simulink model "blockModel"  (R2019b)
settings: Solver=VariableStepAuto  StartTime=0.0  StopTime=10.0  RelTol=1e-3
undefined symbols (not defined in the file or in its folder): gearbox, motor, tyre, veh
libraries: dspsigops x1
settings Model: Creator=picku  LastModifiedBy=picku

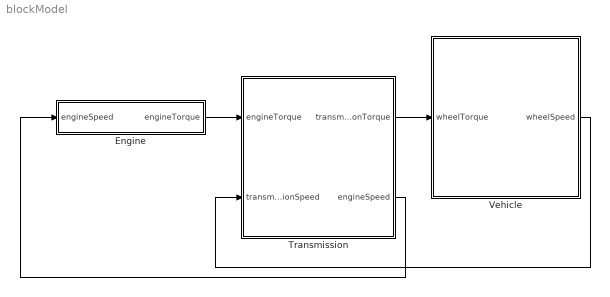
== system blockModel ==
  "Engine " : Subsystem
  Transmission : Subsystem
  Vehicle : Subsystem
  wires:
  Vehicle/1(wheelSpeed) -> Transmission/2(transmissionSpeed)
  Transmission/1(transmissionTorque) -> Vehicle/1(wheelTorque)
  "Engine "/1(engineTorque) -> Transmission/1("engineTorque ")
  Transmission/2(engineSpeed) -> "Engine "/1(engineSpeed)

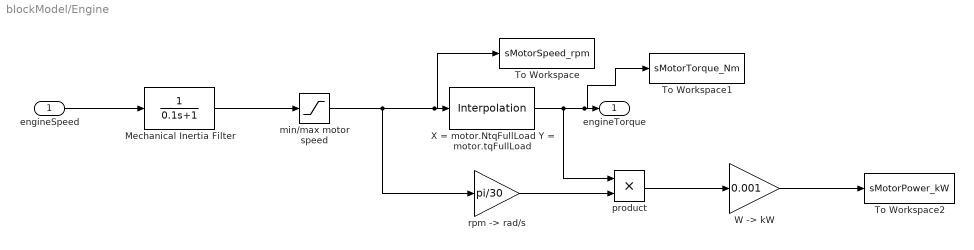
== system blockModel/Engine  ==
  engineSpeed : Inport
  Mechanical Inertia Filter : TransferFcn  Denominator=[0.1 1]
  To Workspace : ToWorkspace  VariableName=sMotorSpeed_rpm  SaveFormat=Timeseries  SampleTime=-1
  To Workspace1 : ToWorkspace  VariableName=sMotorTorque_Nm  SaveFormat=Timeseries  SampleTime=-1
  To Workspace2 : ToWorkspace  VariableName=sMotorPower_kW  SaveFormat=Timeseries  SampleTime=-1
  "W -> kW" : Gain  Gain=0.001
  X = motor.NtqFullLoad Y = motor.tqFullLoad : dspsigops/Interpolation  InterpSource=Specify via dialog  InterpPoints=[motor.NtqFullLoad' motor.tqFullLoad']  InterpMode=Linear  InterpL=3  InterpR=3  InterpAlpha=0.5  InvalidMode=Clip
      settings: SourceProductName=DSP System Toolbox  SourceProductBaseCode=DS
  min/max motor speed : Saturate  UpperLimit=motor.Nmax  LowerLimit=motor.Nmin
  product : Product
  "rpm -> rad/s" : Gain  Gain=pi/30
  engineTorque : Outport
  wires:
  min/max motor speed/1 -> X = motor.NtqFullLoad Y = motor.tqFullLoad/1, To Workspace/1, "rpm -> rad/s"/1
  X = motor.NtqFullLoad Y = motor.tqFullLoad/1 -> To Workspace1/1, engineTorque/1, product/1
  product/1 -> "W -> kW"/1
  "W -> kW"/1 -> To Workspace2/1
  Mechanical Inertia Filter/1 -> min/max motor speed/1
  "rpm -> rad/s"/1 -> product/2
  engineSpeed/1 -> Mechanical Inertia Filter/1

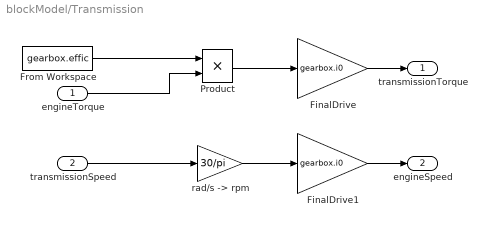
== system blockModel/Transmission ==
  "engineTorque " : Inport
  transmissionSpeed : Inport  Port=2
  FinalDrive : Gain  Gain=gearbox.i0
  FinalDrive1 : Gain  Gain=gearbox.i0
  From Workspace : FromWorkspace  VariableName=gearbox.effic  SampleTime=0
  "Product " : Product
  "rad/s -> rpm" : Gain  Gain=30/pi
  transmissionTorque : Outport
  engineSpeed : Outport  Port=2
  wires:
  "Product "/1 -> FinalDrive/1
  FinalDrive1/1 -> engineSpeed/1
  From Workspace/1 -> "Product "/1
  "engineTorque "/1 -> "Product "/2
  FinalDrive/1 -> transmissionTorque/1
  transmissionSpeed/1 -> "rad/s -> rpm"/1
  "rad/s -> rpm"/1 -> FinalDrive1/1

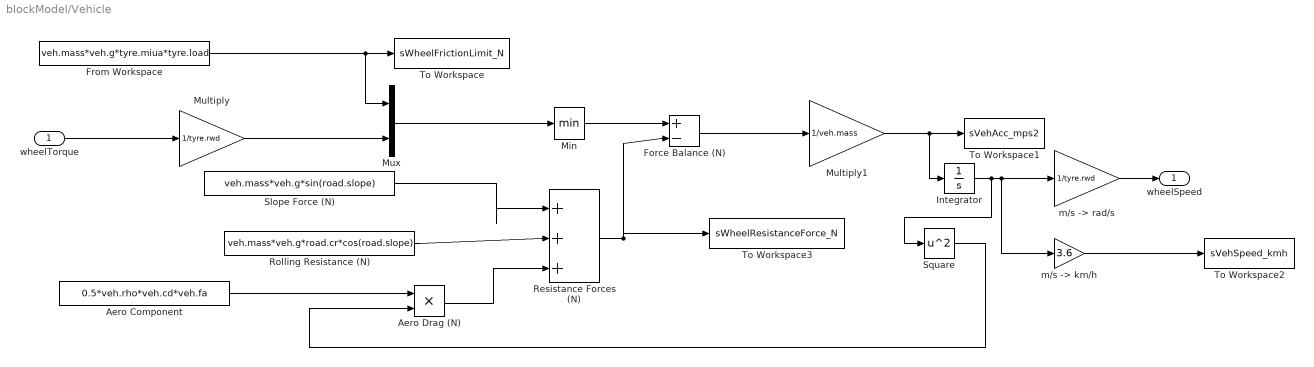
== system blockModel/Vehicle ==
  wheelTorque : Inport
  Aero Component : FromWorkspace  VariableName=0.5*veh.rho*veh.cd*veh.fa  SampleTime=0
  Aero Drag (N) : Product
  Force Balance (N) : Sum  Inputs=+-
  From Workspace : FromWorkspace  VariableName=veh.mass*veh.g*tyre.miua*tyre.load  SampleTime=0
  "Integrator " : Integrator
  Min : MinMax
  Multiply : Gain  Gain=1/tyre.rwd
  Multiply1 : Gain  Gain=1/veh.mass
  Mux : Mux  Inputs=2
  Resistance Forces (N) : Sum  Inputs=|+++
  Rolling Resistance (N) : FromWorkspace  VariableName=veh.mass*veh.g*road.cr*cos(road.slope)  SampleTime=0
  Slope Force (N) : FromWorkspace  VariableName=veh.mass*veh.g*sin(road.slope)  SampleTime=0
  Square : Math  Operator=square  SignedPower=off  SaturateOnIntegerOverflow=on
  To Workspace : ToWorkspace  VariableName=sWheelFrictionLimit_N  SaveFormat=Timeseries  SampleTime=-1
  To Workspace1 : ToWorkspace  VariableName=sVehAcc_mps2  SaveFormat=Timeseries  SampleTime=-1
  To Workspace2 : ToWorkspace  VariableName=sVehSpeed_kmh  SaveFormat=Timeseries  SampleTime=-1
  To Workspace3 : ToWorkspace  VariableName=sWheelResistanceForce_N  SaveFormat=Timeseries  SampleTime=-1
  "m/s -> km/h" : Gain  Gain=3.6
  "m/s -> rad/s" : Gain  Gain=1/tyre.rwd
  wheelSpeed : Outport
  wires:
  Min/1 -> Force Balance (N)/1
  Mux/1 -> Min/1
  Slope Force (N)/1 -> Resistance Forces (N)/1
  Rolling Resistance (N)/1 -> Resistance Forces (N)/2
  Aero Component/1 -> Aero Drag (N)/1
  Aero Drag (N)/1 -> Resistance Forces (N)/3
  Square/1 -> Aero Drag (N)/2
  From Workspace/1 -> Mux/1, To Workspace/1
  "m/s -> rad/s"/1 -> wheelSpeed/1
  Multiply/1 -> Mux/2
  wheelTorque/1 -> Multiply/1
  "Integrator "/1 -> Square/1, "m/s -> rad/s"/1, "m/s -> km/h"/1
  Force Balance (N)/1 -> Multiply1/1
  "m/s -> km/h"/1 -> To Workspace2/1
  Resistance Forces (N)/1 -> To Workspace3/1, Force Balance (N)/2
  Multiply1/1 -> "Integrator "/1, To Workspace1/1
